simulink model "autopilot_model"  (Simulink 8.1)
settings: Solver=FixedStepDiscrete  StartTime=0.0  StopTime=inf  FixedStep=1/100  RelTol=1e-3
libraries: c280xlib x9, idelinklib_ticcs x1, idelinklib_tgtpref x1
settings Model: Creator=nocs  LastModifiedBy=valeria
settings DataIOCC: SaveOutput=off  SaveTime=off
settings OptimizationCC: OptimizeModelRefInitCode=on  LifeSpan=1
settings HardwareCC: ProdBitPerChar=16  ProdBitPerInt=16  ProdBitPerPointer=16  ProdLargestAtomicInteger=Integer  ProdIntDivRoundTo=Zero  ProdEndianess=LittleEndian  ProdWordSize=16  ProdHWDeviceType=Texas Instruments->C2000
settings RTWCC: SystemTargetFile=idelink_ert.tlc  GenerateMakefile=off  TemplateMakefile=idelink_ert.tmf  Description=Embedded IDE Link ERT  ProcessScript=idelink_ert_make_rtw_hook
settings CodeAppCC: IgnoreCustomStorageClasses=off  CustomSymbolStrType=$N$R$M  InternalIdentifier=Classic
settings ERTFactory: TargetFcnLib=ansi_tfl_table_tmw.mat  CodeReplacementLibrary=ANSI_C  UtilityFuncGeneration=Auto  ERTMultiwordTypeDef=System defined  ERTMultiwordLength=256  MultiwordLength=2048  GenerateFullHeader=on  GenerateSampleERTMain=off  GenerateTestInterfaces=off  IsPILTarget=off  ModelReferenceCompliant=on  ParMdlRefBuildCompliant=off  CompOptLevelCompliant=off  ConcurrentExecutionCompliant=on  IncludeMdlTerminateFcn=on  GeneratePreprocessorConditionals=Disable all  CombineOutputUpdateFcns=on  CombineSignalStateStructs=off  SuppressErrorStatus=off  ERTFirstTimeCompliant=off  IncludeFileDelimiter=Auto  ERTCustomFileBanners=on  SupportAbsoluteTime=on  LogVarNameModifier=rt_  MatFileLogging=off  MultiInstanceERTCode=off  SupportNonFinite=on  SupportComplex=on  PurelyIntegerCode=off  SupportContinuousTime=off  SupportNonInlinedSFcns=off  SupportVariableSizeSignals=off  EnableShiftOperators=on  ParenthesesLevel=Nominal  MATLABClassNameForMDSCustomization=linkfoundation.pjtgenerator.IdelinkCustomization  ModelStepFunctionPrototypeControlCompliant=on  CPPClassGenCompliant=off  AutosarCompliant=off  GRTInterface=off  GenerateAllocFcn=off  GenerateASAP2=off  ExtMode=off  ExtModeTransport=0  ExtModeStaticAlloc=off  ExtModeStaticAllocSize=1000000  ExtModeTesting=off  ExtModeMexFile=TIC2000ExternalModeOpen  ExtModeIntrfLevel=Level2 - Open  InlinedParameterPlacement=Hierarchical  TargetOS=BareBoardExample  MultiInstanceErrorCode=Error  RateGroupingCode=on  RootIOFormat=Individual arguments  RTWCAPISignals=off  RTWCAPIParams=off  RTWCAPIStates=off  RTWCAPIRootIO=off  ERTSrcFileBannerTemplate=ert_code_template.cgt  ERTHdrFileBannerTemplate=ert_code_template.cgt  ERTDataSrcFileTemplate=ert_code_template.cgt  ERTDataHdrFileTemplate=ert_code_template.cgt  ERTCustomFileTemplate=example_file_process.tlc  EnableDataOwnership=off  SignalDisplayLevel=10  ParamTuneLevel=10  GlobalDataDefinition=Auto  DataDefinitionFile=global.c  GlobalDataReference=Auto  ERTFilePackagingFormat=Modular  DataReferenceFile=global.h  PreserveExpressionOrder=off  PreserveIfCondition=off  ConvertIfToSwitch=off  PreserveExternInFcnDecls=on  SuppressUnreachableDefaultCases=off  EnableUserReplacementTypes=off  MemSecPackage=--- None ---  MemSecDataConstants=Default  MemSecDataIO=Default  MemSecDataInternal=Default  MemSecDataParameters=Default  MemSecFuncInitTerm=Default  MemSecFuncExecute=Default  MemSecFuncSharedUtil=Default  AdaptorName=Texas Instruments Code Composer Studio v4 (makefile generation only)  exportIDEObj=on  ideObjName=IDE_Obj  oldideObjName=IDE_Obj  ideObjTimeout=10  oldideObjTimeout=10  ideObjBuildTimeout=1000  oldideObjBuildTimeout=1000  TargetPrefTimeStamp=01-Mar-2015 14:34:26  ProfileGenCode=off  profileBy=Tasks  ProfileNumSamples=100  InlineDSPBlks=off  projectOptions=Custom  debugCompilerOptions="-g -D\"_DEBUG\""  releaseCompilerOptions=-o2  getCompilerOptions=off  resetCompilerOptions=off  getLinkerOptions=off  resetLinkerOptions=off  systemStackSize=512  systemHeapSize=512  buildFormat=Makefile  buildAction=Build_and_execute  overrunNotificationMethod=None  overrunNotificationFcn=myfunction  oldoverrunNotificationFcn=myfunction  configurePIL=off  configPILBlockAction=Create_PIL_block_build_and_download  TargetResourceManagerActiveTab=0  DiagnosticActions=warning
settings TargetHardwareResources: Description=Target Hardware Resources Component
settings MATStruct: cache=[]  boardType=F28335 eZdsp  isSimulator=[0.0]  enableHSRTDX=[0.0]  versionNumber=2.9.1  enableDSPBIOSTab=[0.0]  RTOS=None  procName=CPU  boardName=F2812 Device Simulator  realtimesupport=on  tag=ccslinktgtpref_ccsv4  deviceID=F28335  subFamily=2833x  cpuClockRateMHz=[150.0]  codegenhookpoint=C2000  mvSwitch=-v28 --float_support=fpu32  numSections=[23.0]  numRTOS=[1.0]  defaultSysStackSize=[512.0]  isBuiltIn=[1]  numBanks=[16.0]  numCacheLvl=[0.0]  isremovable=[0.0]  iscontentsfixed=[0.0]  name=BEGINRAM  addr=[0.0]  size=[2.0]  contents=Code  space=Internal  createHeap=[0.0]  heapSize=[256.0]  defineLabel=[0.0]  heapLabel=segment_name  label=None  timer=[]  timerprescaler=[]  description=C code  codeObjectMem=IPRAM  dataObjectMem=IDRAM  section=[]  enable=off  schedulerType=Rate priority  stackSize=[4096.0]  staticStackMemSegment=IDRAM  dynamicStackMemSegment=MEM_NULL  errId=[]  DSPChipLabel=TI TMS320C28335  ADCLKPS=3  CPS=1  ACQ_PS=4  OffsetCorrectionValue=[0.0]  ExternalReferenceSelector=off  Continuous=off  ADCCLK=[6.25]  AcquisitionWindow=[0.8]  BaudRatePrescaler=[5.0]  TSEG1=8  TSEG2=6  SBG=Only_falling_edges  SJW=2  SAM=Sample_one_time  EnhancedCANMode=on  SelfTestMode=off  PinAssignment_Tx=GPIO31  PinAssignment_Rx=GPIO30  ModuleClockFrequency=[75.0]  BaudRate=[1000000.0]  PinAssignment_ECAP1=GPIO5  PinAssignment_ECAP2=GPIO7  PinAssignment_ECAP3=GPIO9  PinAssignment_ECAP4=GPIO11  PinAssignment_ECAP5=GPIO3  PinAssignment_ECAP6=GPIO1  PinAssignment_SYNCI=None  PinAssignment_SYNCO=None  Mode=Master  AddrDataFormat=7-Bit Addressing  OwnAddress=[1.0]  BitCount=8  MasterClockFrequency=[750000.0]  ModuleClockPrescaler=[9.0]  MasterClkLowTime=[5.0]  MasterClkHighTime=[5.0]  EnableLoopback=off  EnableTxInt=off  TxFifoLevel=0  EnableRxInt=off  RxFifoLevel=0  EnableSysInt=off  AAS=off  SCD=off  ARDY=off  NACK=off  AL=off  EnableLoopBack=off  SuspensionMode=Free_run  NumberOfStopBits=1  ParityMode=None  CharacterLengthBits=8  CommunicationMode=Raw_data  BlockingMode=off  DataByteOrder=Little_Endian  DataSwapWidth=8_bits  UserBaudRate=115200  BaudRateFactor=[127.0]  DataBits=16  ClockPolarity=Rising_edge  ClockPhase=No_delay  FIFOEnable=off  FIFOInterruptLevel_Rx=16  FIFOInterruptLevel_Tx=0  FIFOTransmitDelay=[0.0]  PinAssignment_CLK=GPIO18  PinAssignment_SOMI=GPIO17  PinAssignment_STE=GPIO19  PinAssignment_SIMO=GPIO16  PinAssignment_eQEP1A=GPIO20  PinAssignment_eQEP1B=GPIO21  PinAssignment_eQEP1S=GPIO22  PinAssignment_eQEP1I=GPIO23  Enable_watchdog=off  Watchdogclock=OSCCLK/512/1  Time_period=[0.0043690666666666668]  Watchdogevent=Chip reset  QualPRD=[0.0]  GPIOQualSel0=Synchronize to SYSCLKOUT only  GPIOQualSel1=Synchronize to SYSCLKOUT only  GPIOQualSel2=Synchronize to SYSCLKOUT only  GPIOQualSel3=Synchronize to SYSCLKOUT only  GPIOQualSel4=Synchronize to SYSCLKOUT only  GPIOQualSel5=Synchronize to SYSCLKOUT only  GPIOQualSel6=Synchronize to SYSCLKOUT only  GPIOQualSel7=Synchronize to SYSCLKOUT only  GPIOQualSel8=Synchronize to SYSCLKOUT only  GPIOQualSel9=Synchronize to SYSCLKOUT only  GPIOQualSel10=Synchronize to SYSCLKOUT only  GPIOQualSel11=Synchronize to SYSCLKOUT only  GPIOQualSel12=Synchronize to SYSCLKOUT only  GPIOQualSel13=Synchronize to SYSCLKOUT only  GPIOQualSel14=Synchronize to SYSCLKOUT only  GPIOQualSel15=Synchronize to SYSCLKOUT only  GPIOQualSel16=Synchronize to SYSCLKOUT only  GPIOQualSel17=Synchronize to SYSCLKOUT only  GPIOQualSel18=Synchronize to SYSCLKOUT only  GPIOQualSel19=Synchronize to SYSCLKOUT only  GPIOQualSel20=Synchronize to SYSCLKOUT only  GPIOQualSel21=Synchronize to SYSCLKOUT only  GPIOQualSel22=Synchronize to SYSCLKOUT only  GPIOQualSel23=Synchronize to SYSCLKOUT only  GPIOQualSel24=Synchronize to SYSCLKOUT only  GPIOQualSel25=Synchronize to SYSCLKOUT only  GPIOQualSel26=Synchronize to SYSCLKOUT only  GPIOQualSel27=Synchronize to SYSCLKOUT only  GPIOQualSel28=Synchronize to SYSCLKOUT only  GPIOQualSel29=Synchronize to SYSCLKOUT only  GPIOQualSel30=Synchronize to SYSCLKOUT only  GPIOQualSel31=Synchronize to SYSCLKOUT only  GPIOQualSel32=Synchronize to SYSCLKOUT only  GPIOQualSel33=Synchronize to SYSCLKOUT only  GPIOQualSel34=Synchronize to SYSCLKOUT only  GPIOQualSel35=Synchronize to SYSCLKOUT only  GPIOQualSel36=Synchronize to SYSCLKOUT only  GPIOQualSel37=Synchronize to SYSCLKOUT only  GPIOQualSel38=Synchronize to SYSCLKOUT only  GPIOQualSel39=Synchronize to SYSCLKOUT only  GPIOQualSel40=Synchronize to SYSCLKOUT only  GPIOQualSel41=Synchronize to SYSCLKOUT only  GPIOQualSel42=Synchronize to SYSCLKOUT only  GPIOQualSel43=Synchronize to SYSCLKOUT only  GPIOQualSel44=Synchronize to SYSCLKOUT only  GPIOQualSel45=Synchronize to SYSCLKOUT only  GPIOQualSel46=Synchronize to SYSCLKOUT only  GPIOQualSel47=Synchronize to SYSCLKOUT only  GPIOQualSel48=Synchronize to SYSCLKOUT only  GPIOQualSel49=Synchronize to SYSCLKOUT only  GPIOQualSel50=Synchronize to SYSCLKOUT only  GPIOQualSel51=Synchronize to SYSCLKOUT only  GPIOQualSel52=Synchronize to SYSCLKOUT only  GPIOQualSel53=Synchronize to SYSCLKOUT only  GPIOQualSel54=Synchronize to SYSCLKOUT only  GPIOQualSel55=Synchronize to SYSCLKOUT only  GPIOQualSel56=Synchronize to SYSCLKOUT only  GPIOQualSel57=Synchronize to SYSCLKOUT only  GPIOQualSel58=Synchronize to SYSCLKOUT only  GPIOQualSel59=Synchronize to SYSCLKOUT only  GPIOQualSel60=Synchronize to SYSCLKOUT only  GPIOQualSel61=Synchronize to SYSCLKOUT only  GPIOQualSel62=Synchronize to SYSCLKOUT only  GPIOQualSel63=Synchronize to SYSCLKOUT only  Enable_Flash=Disable  Automatic=on  SectorA=on  SectorB=on  SectorC=on  SectorD=on  SectorE=on  SectorF=on  SectorG=on  SectorH=on  SectorI=on  SectorJ=on  APIBrowse=Browse  API_Dir=C:\tidcs\c28\Flash28_API\Flash28335_API_V101\lib\Flash28335_API_V101.lib  Execute=Execute  EnableDMAChannel=off  DataSize=16 bit  InterruptSrc=None  ExternalPin=0  BurstSize=1  TransferSize=1  WrapSrcSize=65536  WrapDstSize=65536  SrcBeginAdd=0xC000  SrcBurstStep=0  SrcTransStep=0  SrcWrapStep=0  DstBeginAdd=0xD000  DstBurstStep=0  DstTransStep=0  DstWrapStep=0  GenInterrupt=Never  EnableOneShot=off  SyncEnable=off  EnableContinuous=off  EnableDSTSync=off  SetCh1ToHigh=off  EnableOverFlow=off  OSCCLK=[30.0]  AutoSetPllSettings=on  PLLCR=10  DIVSEL=(OSCCLK * PLLCR)/2  ClosestCpuClock=[150.0]  LspclkDiv=SYSCLKOUT/4  LSPCLK=[37.5]  HspclkDiv=SYSCLKOUT/2  HSPCLK=[75.0]  schedulingMode=real-time  baseRatePriority=[40.0]

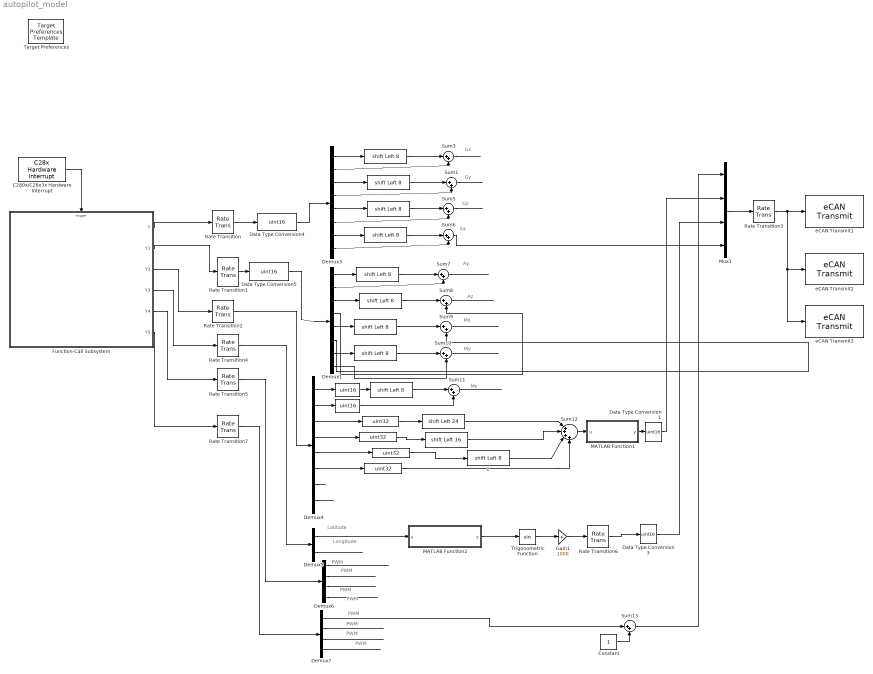
== system autopilot_model ==
  note: Ay
  note: Ax
  note: Gy
  note: Gx
  note: Gz
  note: Az
  note: Mx
  note: My
  note: Mz
  note: PWM
  note: PWM
  note: PWM
  note: PWM
  note: Latitude
  note: Longitude
  note: PWM
  note: PWM
  note: PWM
  note: PWM
  " " : ArithShift  BitShiftNumber=24  BitShiftDirection=Left
  "  " : ArithShift  BitShiftNumber=16  BitShiftDirection=Left
  "    " : ArithShift  BitShiftNumber=8  BitShiftDirection=Left
  "     " : ArithShift  BitShiftNumber=8  BitShiftDirection=Left
  "      " : DataTypeConversion  OutDataTypeStr=uint32
  "        " : ArithShift  BitShiftNumber=8  BitShiftDirection=Left
  "            " : ArithShift  BitShiftNumber=8  BitShiftDirection=Left
  "                   " : ArithShift  BitShiftNumber=8  BitShiftDirection=Left
  "                              " : ArithShift  BitShiftNumber=8  BitShiftDirection=Left
  "                                   " : ArithShift  BitShiftNumber=8  BitShiftDirection=Left
  "                                          " : DataTypeConversion  OutDataTypeStr=uint32
  "                                                " : ArithShift  BitShiftNumber=8  BitShiftDirection=Left
  "                                                   " : DataTypeConversion  OutDataTypeStr=uint32
  "                                                          " : ArithShift  BitShiftNumber=8  BitShiftDirection=Left
  "                                                                           " : DataTypeConversion  OutDataTypeStr=uint32
  "                                                                                                                " : DataTypeConversion  OutDataTypeStr=uint16
  "                                                                                                                                         " : DataTypeConversion  OutDataTypeStr=uint16
  "  2" : ArithShift  BitShiftNumber=8  BitShiftDirection=Left
  C280x/C28x3x Hardware Interrupt : idelinklib_ticcs/C28x Hardware Interrupt  irqnumbers=[9]  pienumbers=[5]  irqpriorities=[30]  irqpreempts=[0]  showinput=off  dspchiptype=C280X
  Constant : Constant  OutDataTypeStr=uint16
  Data Type Conversion{1,3..5} (4 alike) : DataTypeConversion  OutDataTypeStr=uint16
  Demux1 : Demux  Outputs=8
  Demux3 : Demux  Outputs=8
  Demux4 : Demux  Outputs=8
  Demux5 : Demux  Outputs=2
  Demux6 : Demux
  Demux7 : Demux
  Function-Call Subsystem : Subsystem  TreatAsAtomicUnit=on
  Gain1 : Gain  Gain=1000
  MATLAB Function1 : MATLAB Function  TreatAsAtomicUnit=on
      settings: RTWSystemCode=Inline
  MATLAB Function2 : MATLAB Function  TreatAsAtomicUnit=on
      settings: RTWSystemCode=Inline
  Mux1 : Mux
  Rate Transition{,1..2,4..7} (7 alike) : RateTransition  Deterministic=off
  Rate Transition3 : RateTransition  Deterministic=off  OutPortSampleTime=0.01
  Sum{1,3,5..11,13} (10 alike) : Sum  Inputs=|++
  Sum12 : Sum  Inputs=|++++
  Target Preferences : idelinklib_tgtpref/Target Preferences Template  Tag=ccslinktgtpref_ccsv4  library=off
  Trigonometric Function : Trigonometry
  eCAN Transmit1 : c280xlib/eCAN Transmit  chipFamily=C28x3x  useModule=eCAN_A  mailboxNo=2  messageID=bin2dec('10100001111')  messageType=Standard (11-bit identifier)  enableBlockingMode=off  postInterrupt=off  interruptLine=0
  eCAN Transmit2 : c280xlib/eCAN Transmit  chipFamily=C28x3x  useModule=eCAN_A  mailboxNo=13  messageID=bin2dec('10100011111')  messageType=Standard (11-bit identifier)  enableBlockingMode=off  postInterrupt=off  interruptLine=0
  eCAN Transmit3 : c280xlib/eCAN Transmit  chipFamily=C28x3x  useModule=eCAN_A  mailboxNo=12  messageID=bin2dec('10100101111')  messageType=Standard (11-bit identifier)  enableBlockingMode=off  postInterrupt=off  interruptLine=0
  wires:
  C280x/C28x3x Hardware Interrupt/1 -> Function-Call Subsystem/Trigger
  Function-Call Subsystem/1(Y) -> Rate Transition/1
  Function-Call Subsystem/2(Y1) -> Rate Transition1/1
  Function-Call Subsystem/3(Y2) -> Rate Transition2/1
  Function-Call Subsystem/4(Y3) -> Rate Transition4/1
  Function-Call Subsystem/5(Y4) -> Rate Transition5/1
  Rate Transition3/1 -> eCAN Transmit1/1, eCAN Transmit2/1, eCAN Transmit3/1
  Rate Transition1/1 -> Data Type Conversion5/1
  "    "/1 -> Sum3/1
  Demux3/2 -> Sum3/2
  Demux3/1 -> "    "/1
  Mux1/1 -> Rate Transition3/1
  Rate Transition/1 -> Data Type Conversion4/1
  Data Type Conversion4/1 -> Demux3/1
  Data Type Conversion5/1 -> Demux1/1
  "     "/1 -> Sum1/1
  Demux3/4 -> Sum1/2
  Demux3/3 -> "     "/1
  "        "/1 -> Sum5/1
  Demux3/5 -> "        "/1
  Demux3/6 -> Sum5/2
  "                                   "/1 -> Sum6/1
  Demux3/8 -> Sum6/2
  Demux3/7 -> "                                   "/1
  Sum1/1 -> ?
  Sum5/1 -> ?
  "                                                          "/1 -> Sum7/1
  Demux1/2 -> Sum7/2
  Demux1/1 -> "                                                          "/1
  Sum7/1 -> ?
  Sum6/1 -> Mux1/4
  Demux1/3 -> "                                                "/1
  "                                                "/1 -> Sum8/1
  Demux1/4 -> Sum8/2
  Sum8/1 -> ?
  Demux1/5 -> "                   "/1
  "                   "/1 -> Sum9/1
  Demux1/6 -> Sum9/2
  Sum9/1 -> ?
  Demux1/7 -> "            "/1
  "            "/1 -> Sum10/1
  Demux1/8 -> Sum10/2
  Sum10/1 -> ?
  Rate Transition2/1 -> Demux4/1
  Demux4/1 -> "                                                                                                                "/1
  "                              "/1 -> Sum11/1
  Demux4/2 -> "                                                                                                                                         "/1
  Sum11/1 -> ?
  Demux4/3 -> "                                                   "/1
  Demux4/4 -> "      "/1
  Demux4/5 -> "                                          "/1
  "                                                   "/1 -> " "/1
  Demux4/6 -> "                                                                           "/1
  "                                                                                                                "/1 -> "                              "/1
  "                                                                                                                                         "/1 -> Sum11/2
  "      "/1 -> "  "/1
  "                                          "/1 -> "  2"/1
  "  "/1 -> Sum12/2
  "  2"/1 -> Sum12/3
  "                                                                           "/1 -> Sum12/4
  " "/1 -> Sum12/1
  Sum12/1 -> MATLAB Function1/1(u)
  Demux4/7 -> ?
  Demux4/8 -> ?
  Rate Transition4/1 -> Demux5/1
  Function-Call Subsystem/6(Y5) -> Rate Transition7/1
  Rate Transition5/1 -> Demux6/1
  Rate Transition7/1 -> Demux7/1
  Demux5/2 -> ?
  Demux6/2 -> ?
  Demux6/3 -> ?
  Demux6/4 -> ?
  Demux7/2 -> ?
  Demux7/3 -> ?
  Demux7/4 -> ?
  MATLAB Function1/1(y) -> Data Type Conversion1/1
  Data Type Conversion1/1 -> Mux1/2
  Demux6/1 -> ?
  MATLAB Function2/1(y) -> Trigonometric Function/1
  Trigonometric Function/1 -> Gain1/1
  Demux5/1 -> MATLAB Function2/1(u)
  Gain1/1 -> Rate Transition6/1
  Data Type Conversion3/1 -> Mux1/3
  Rate Transition6/1 -> Data Type Conversion3/1
  Sum3/1 -> ?
  Demux7/1 -> Sum13/1
  Sum13/1 -> Mux1/1
  Constant/1 -> Sum13/2

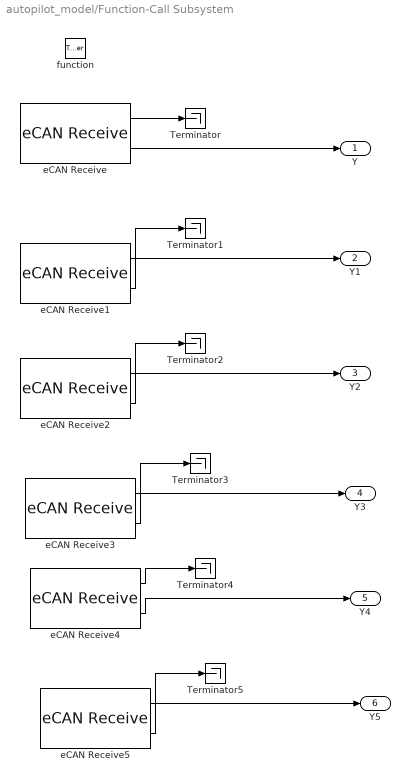
== system autopilot_model/Function-Call Subsystem ==
  function : TriggerPort  TriggerType=function-call
  Terminator{,1..5} (6 alike) : Terminator
  eCAN Receive : c280xlib/eCAN Receive  chipFamily=C28x3x  useModule=eCAN_A  mailboxNo=0  messageID=bin2dec('11000001111')  messageType=Standard (11-bit identifier)  sampleTime=-1  dataType=uint8  initValue=0  outputMessageLength=off  outputMessageTimeStamp=off  postInterrupt=on  interruptLine=0
  eCAN Receive1 : c280xlib/eCAN Receive  chipFamily=C28x3x  useModule=eCAN_A  mailboxNo=3  messageID=bin2dec('10000001111')  messageType=Standard (11-bit identifier)  sampleTime=-1  dataType=uint8  initValue=0  outputMessageLength=off  outputMessageTimeStamp=off  postInterrupt=on  interruptLine=0
  eCAN Receive2 : c280xlib/eCAN Receive  chipFamily=C28x3x  useModule=eCAN_A  mailboxNo=4  messageID=bin2dec('01100001111')  messageType=Standard (11-bit identifier)  sampleTime=-1  dataType=uint8  initValue=0  outputMessageLength=off  outputMessageTimeStamp=off  postInterrupt=on  interruptLine=0
  eCAN Receive3 : c280xlib/eCAN Receive  chipFamily=C28x3x  useModule=eCAN_A  mailboxNo=7  messageID=bin2dec('01000001111')  messageType=Standard (11-bit identifier)  sampleTime=-1  dataType=uint32  initValue=0  outputMessageLength=off  outputMessageTimeStamp=off  postInterrupt=on  interruptLine=0
  eCAN Receive4 : c280xlib/eCAN Receive  chipFamily=C28x3x  useModule=eCAN_A  mailboxNo=8  messageID=bin2dec('00100001111')  messageType=Standard (11-bit identifier)  sampleTime=-1  dataType=uint16  initValue=0  outputMessageLength=off  outputMessageTimeStamp=off  postInterrupt=on  interruptLine=0
  eCAN Receive5 : c280xlib/eCAN Receive  chipFamily=C28x3x  useModule=eCAN_A  mailboxNo=10  messageID=bin2dec('11100001111')  messageType=Standard (11-bit identifier)  sampleTime=-1  dataType=uint16  initValue=0  outputMessageLength=off  outputMessageTimeStamp=off  postInterrupt=on  interruptLine=0
  Y : Outport
  Y1 : Outport  Port=2
  Y2 : Outport  Port=3
  Y3 : Outport  Port=4
  Y4 : Outport  Port=5
  Y5 : Outport  Port=6
  wires:
  eCAN Receive/2 -> Y/1
  eCAN Receive/1 -> Terminator/1
  eCAN Receive1/2 -> Y1/1
  eCAN Receive1/1 -> Terminator1/1
  eCAN Receive2/2 -> Y2/1
  eCAN Receive2/1 -> Terminator2/1
  eCAN Receive3/2 -> Y3/1
  eCAN Receive3/1 -> Terminator3/1
  eCAN Receive4/2 -> Y4/1
  eCAN Receive4/1 -> Terminator4/1
  eCAN Receive5/2 -> Y5/1
  eCAN Receive5/1 -> Terminator5/1

== matlab function MATLAB Function1 ==
  data: u input uint32; y output single
function y = fcn_unit322single(u)
%#codegen

y = typecast(u,'single');

== matlab function MATLAB Function2 ==
  data: u input uint32; y output single
function y = fcn_unit322single(u)
%#codegen

y = typecast(u,'single');
